simulink model "Exp_3_batch_17_Simulation (4)"  (R2020a)
settings: Solver=VariableStepAuto  StartTime=0.0  StopTime=20  RelTol=1e-3
settings Model: Creator=sundaram bhupathi  LastModifiedBy=tarun

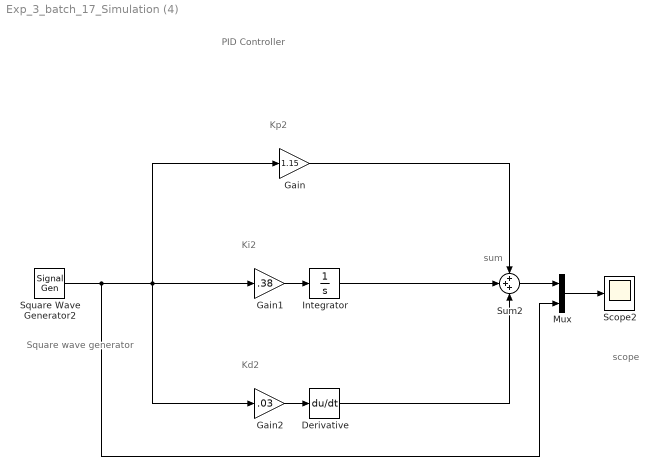
== system Exp_3_batch_17_Simulation (4) ==
  note: Kd2
  note: Ki2
  note: Kp2
  note: PID Controller
  note: sum
  note: scope
  note: Square wave generator
  Derivative : Derivative
  Gain : Gain  Gain=1.15
  Gain1 : Gain  Gain=.38
  Gain2 : Gain  Gain=.03
  Integrator : Integrator
  Mux : Mux  Inputs=2
  Scope2 : Scope
  Square Wave Generator2 : SignalGenerator  WaveForm=square  Amplitude=10  Units=rad/sec
  Sum2 : Sum  Inputs=+++  InputSameDT=on  SaturateOnIntegerOverflow=on  OutDataTypeStr=Inherit: Same as first input
  wires:
  Derivative/1 -> Sum2/3
  Gain/1 -> Sum2/1
  Integrator/1 -> Sum2/2
  Sum2/1 -> Mux/1
  Mux/1 -> Scope2/1
  Gain1/1 -> Integrator/1
  Gain2/1 -> Derivative/1
  Square Wave Generator2/1 -> Gain1/1, Gain2/1, Gain/1, Mux/2
